simulink model "Simulation_Block_Diagram_Battery"  (R2015b)
settings: Solver=ode1  StartTime=0.0  StopTime=43200  FixedStep=0.1  RelTol=1e-3
undefined symbols (not defined in the file): C_1, N_p, N_s, Param, Q_cap, R_0, R_1
settings Model: Creator=Kane Chew  LastModifiedBy=Kane Chew

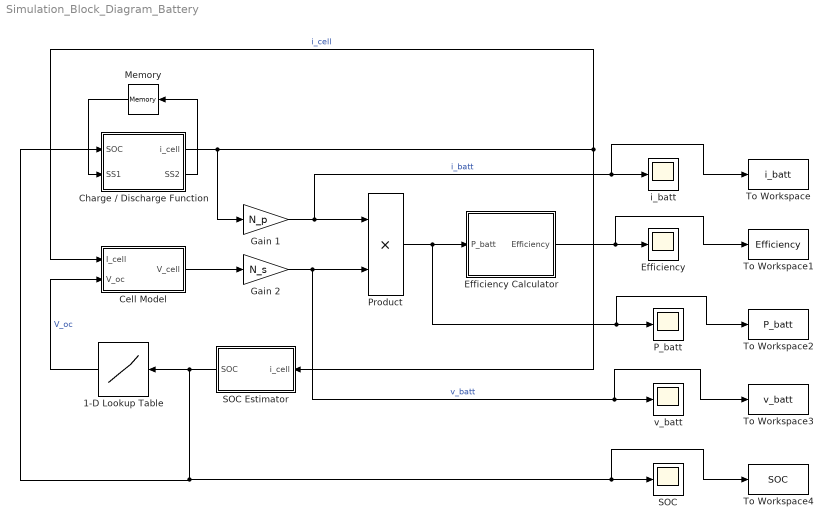
== system Simulation_Block_Diagram_Battery ==
  1-D Lookup Table : Lookup_n-D  NumberOfTableDimensions=1  BreakpointsForDimension1="[0     , 0.10 , 0.25 , 0.50  , 0.75 , 0.90 , 1.00]"  Table=[3.51 , 3.57 , 3.63 , 3.71 , 3.93 , 4.08 , 4.19]  InternalRulePriority=Speed  RndMeth=Simplest  InputSameDT=on
  Cell Model : Subsystem
  Charge / Discharge Function : MATLAB Function  TreatAsAtomicUnit=on
  Efficiency : Scope
  "Efficiency Calculator " : Subsystem
  Gain 1 : Gain  Gain=N_p
  Gain 2 : Gain  Gain=N_s
  Memory : Memory  X0=-1
  P_batt : Scope
  Product : Product  Inputs=**
  SOC : Scope
  SOC Estimator : Subsystem
  To Workspace : ToWorkspace  VariableName=i_batt  SaveFormat=Timeseries  SampleTime=-1
  To Workspace1 : ToWorkspace  VariableName=Efficiency  SaveFormat=Timeseries  SampleTime=-1
  To Workspace2 : ToWorkspace  VariableName=P_batt  SaveFormat=Timeseries  SampleTime=-1
  To Workspace3 : ToWorkspace  VariableName=v_batt  SaveFormat=Timeseries  SampleTime=-1
  To Workspace4 : ToWorkspace  VariableName=SOC  SaveFormat=Timeseries  SampleTime=-1
  i_batt : Scope
  v_batt : Scope
  wires:
  SOC Estimator/1(SOC) -> Charge / Discharge Function/1(SOC), To Workspace4/1, SOC/1, 1-D Lookup Table/1
  1-D Lookup Table/1 -> Cell Model/2(V_oc)  "V_oc"
  Cell Model/1(V_cell) -> Gain 2/1
  Gain 1/1 -> To Workspace/1, i_batt/1, Product/1  "i_batt"
  Gain 2/1 -> To Workspace3/1, v_batt/1, Product/2  "v_batt"
  Charge / Discharge Function/1(i_cell) -> Gain 1/1, Cell Model/1(I_cell), SOC Estimator/1("i_cell ")  "i_cell"
  Charge / Discharge Function/2(SS2) -> Memory/1
  Memory/1 -> Charge / Discharge Function/2(SS1)
  Product/1 -> To Workspace2/1, P_batt/1, "Efficiency Calculator "/1(P_batt)
  "Efficiency Calculator "/1("Efficiency ") -> To Workspace1/1, Efficiency/1

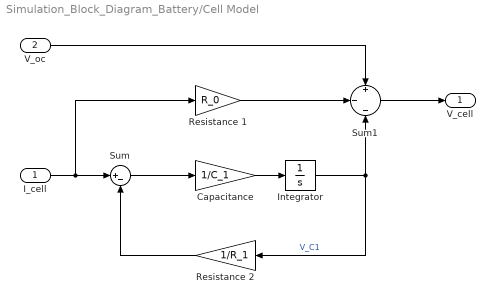
== system Simulation_Block_Diagram_Battery/Cell Model ==
  I_cell : Inport
  V_oc : Inport  Port=2
  Capacitance : Gain  Gain=1/C_1
  Integrator : Integrator
  Resistance 1 : Gain  Gain=R_0
  Resistance 2 : Gain  Gain=1/R_1
  Sum : Sum  Inputs=|+-
  Sum1 : Sum  Inputs=+|-|-
  V_cell : Outport
  wires:
  I_cell/1 -> Resistance 1/1, Sum/1
  Sum/1 -> Capacitance/1
  Capacitance/1 -> Integrator/1
  Resistance 1/1 -> Sum1/2
  Integrator/1 -> Resistance 2/1, Sum1/3  "V_C1"
  Resistance 2/1 -> Sum/2
  V_oc/1 -> Sum1/1
  Sum1/1 -> V_cell/1

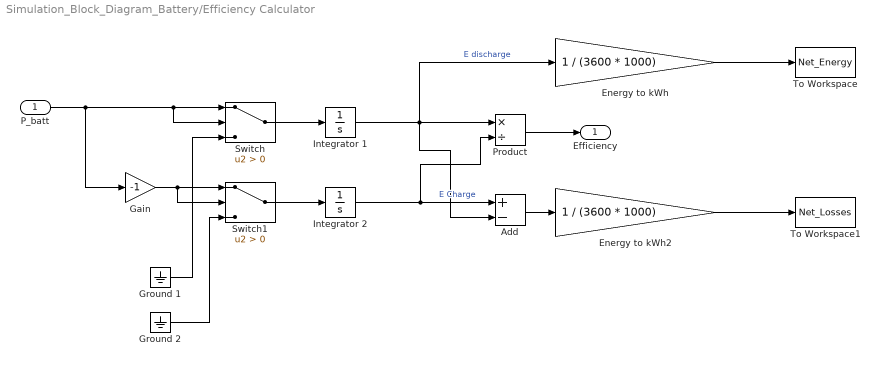
== system Simulation_Block_Diagram_Battery/Efficiency Calculator  ==
  P_batt : Inport
  Add : Sum  Inputs=+-
  Energy to kWh : Gain  Gain=1 / (3600 * 1000)
  Energy to kWh2 : Gain  Gain=1 / (3600 * 1000)
  Gain : Gain  Gain=-1
  Ground 1 : Ground
  Ground 2 : Ground
  Integrator 1 : Integrator
  Integrator 2 : Integrator
  Product : Product  Inputs=*/
  Switch : Switch  Criteria=u2 > Threshold
  Switch1 : Switch  Criteria=u2 > Threshold
  To Workspace : ToWorkspace  VariableName=Net_Energy  SaveFormat=Timeseries  SampleTime=-1
  To Workspace1 : ToWorkspace  VariableName=Net_Losses  SaveFormat=Timeseries  SampleTime=-1
  "Efficiency " : Outport
  wires:
  Integrator 1/1 -> Energy to kWh/1, Add/2, Product/1  "E discharge"
  Integrator 2/1 -> Add/1, Product/2  "E Charge"
  Ground 2/1 -> Switch1/3
  Ground 1/1 -> Switch/3
  P_batt/1 -> Gain/1, Switch/2, Switch/1
  Gain/1 -> Switch1/2, Switch1/1
  Product/1 -> "Efficiency "/1
  Switch/1 -> Integrator 1/1
  Switch1/1 -> Integrator 2/1
  Add/1 -> Energy to kWh2/1
  Energy to kWh/1 -> To Workspace/1
  Energy to kWh2/1 -> To Workspace1/1

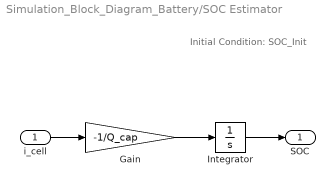
== system Simulation_Block_Diagram_Battery/SOC Estimator ==
  note: Initial Condition:
      | SOC_Init
  "i_cell " : Inport
  Gain : Gain  Gain=-1/Q_cap
  Integrator : Integrator  InitialCondition=Param.SOC_Init
  SOC : Outport
  wires:
  Integrator/1 -> SOC/1
  Gain/1 -> Integrator/1
  "i_cell "/1 -> Gain/1

== matlab function Simulation_Block_Diagram_Battery/Charge // Discharge Function ==
  data: SOC input; i_cell output; SS1 input; SS2 output; Param parameter
function [i_cell,SS2] = fcn(SOC, SS1, Param)

SS2 = SS1;

Cell_C      = Param.Cell_C;
C_rate_c    = Param.C_rate_c;
C_rate_dc   = Param.C_rate_dc;

SOC_Init    = Param.SOC_Init;
SOC_Max     = Param.SOC_Max;

if (SOC <= SOC_Init)
    i_cell = (SS2)* C_rate_c * Cell_C;   % Negative Current charges battery
    SS2 = -1;
    
elseif (SOC < SOC_Max && SOC >SOC_Init && SS2 == -1) % Charging State
    
    i_cell = (SS2)* C_rate_c * Cell_C;  % Maintain Charging Current
            
elseif (SOC < SOC_Max && SOC >SOC_Init && SS2 == 1) % Discharging State
    
    i_cell = (SS2)* C_rate_dc * Cell_C;  % Maintain Dischargig Current
            
elseif (SOC >= SOC_Max)
    
    i_cell = (SS2)* C_rate_dc * Cell_C; % Positive Current discharges battery
    SS2 = 1;
else
    i_cell = 0;                 
end

i_cell;
